simulink model "CM13_2024a_MachE_for_UA_HIL"  (R2024a)
settings: Solver=ode1  StartTime=0.0  StopTime=Inf  FixedStep=0.001  RelTol=1e-3  EnableMultiTasking=on
PreLoadFcn:
  | % if ~length(which('cmcmd')), cmenv; end
PostLoadFcn:
  | if any(exist('dsrtsu_mdlpostloadfcn', 'file') ~= 0), dsrtsu_mdlpostloadfcn('Execute', bdroot); end
InitFcn:
  | , if any(exist('rtifpga_mdlclblib', 'file') ~= 0), rtifpga_mdlclblib('Init', bdroot); end,
  | , if any(exist('dsmpb_private', 'file') ~= 0), dsmpb_private('dsmpb_mdlclblib', 'Init', bdroot); end,
values from neighbouring files (symbols this model uses):
  CoastDown =     [Run_Simulink.mat]
  limitedMCT =     [Run_Simulink.mat]
  MCT =     [Run_Simulink.mat]
  pMCT =     [Run_Simulink.mat]
  RealSimPara =     [Run_Simulink.mat]
  Ref_speed = [13 13.007895099 13.015778396 13.023649891 13.031509584 13.039357475 13.047193564 13.055017851 13.062830336 13.070631019 13.0784199 13.086196979 ... (2669 elements, 2669x1)]    [Ref_speed_and_time.mat]
  Ref_time = [0 0.01 0.02 0.03 0.04 0.05 0.06 0.07 0.08 0.09 0.1 0.11 ... (2669 elements, 2669x1)]    [Ref_speed_and_time.mat]
  US06 =     [Run_Simulink.mat]
undefined symbols (not defined in the file or in its folder): AccelCmd, ActTqLF_Nm_, ActTqLR_Nm_, ActTqRF_Nm_, ActTqRR_Nm_, BattChargeLimitMaxPwr, BattChargeLimitSocBpts, BattChargeLimitTbl, BattChrgCapcty, BattDischargeLimitSocBpts, BattDischargeLimitTbl, BattDischargeMaxPwr, BattNumCellsParallel, BattNumCellsSeries, BattOpenVoltCapBpts, BattOpenVoltTbl, BattResistSocBpts, BattResistTbl, BattResistTempBpts, BrakeMaxPrs, BrakeMaxTrq, ChassisDistCg2FrontAxle, ChassisDistCg2RearAxle, ChassisVehMass, CltchCmd, DecelCmd, DiffRatio, DiscIntNeverNeededParam, EnvGravCnst, EnvPrs, EnvTemp, FuelSpecificGrav, GearCmd, h, InitStates, lgSw, MtrEffSpdBpts, MtrEffTbl, MtrEffTrqBpts, MtrPwrMax, MtrTrqMax, planned_speed, planned_time, ref_speed, ref_time, rticanmm_blockfcn, rticanmm_initfcn, SteeringCmd, SupvsryCtrlRegenBrkCutOffTbl, SupvsryCtrlRegenSpdBpts, TestScnrioCycleNum, VEH
libraries: simulink x264, VSIGenLib x262, etargetslib x201, dsmpblib x161, CarMaker4SL x142, rtimmsu_dsrtlib x32, vehdynlibtire x24, autolibshared x19, vehdynlibsuspension x14, vehdynlibtirecommon x14, autolibutils x10, VsrLibWheel x8
(part 8 of 48)

== system CM13_2024a_MachE_for_UA_HIL/CarMaker/IPG Vehicle/Rototest and ORNL Interface ==
  note: CM driver = 0
      | Simulink driver = 1
  note: rad/s
  CarTrqT2W : Inport
  UDP Input : Inport  Port=2
  BRAKE_PRESSED : Inport  Port=3
  vehSpeedKph : Inport  Port=4
  1/tireRadius : Gain  Gain=1/0.3232
  ChargingMode : Constant  Value=0
  CmdSpeed (mph) : Constant  Value=0
  Constant : Constant  Value=3000
  DriverSwitch : Constant  Value=0
  DummyPT : Subsystem
  Format CM Powertrain Signals : Subsystem
  From Rototest : Subsystem
  Gain1 : Gain  Commented=on  Gain=3.6
  Get Wheel Spd Cmd Based on Wheel Dynamics : Subsystem
  Multiport Switch : MultiPortSwitch  DataPortOrder=Zero-based contiguous  Inputs=2  zeroidx=on  SaturateOnIntegerOverflow=off  InputSameDT=off
  Multiport Switch1 : MultiPortSwitch  DataPortOrder=Zero-based contiguous  Inputs=2  zeroidx=on  SaturateOnIntegerOverflow=off  InputSameDT=off
  Read CM Dict : CarMaker4SL/Read CM Dict  Commented=on  xname=Car.v  xsync=off  xstime=Continuous
  RotoTrqPreprocess : Subsystem
  Subsystem2 : Subsystem
  Terminator2 : Terminator
  To Rototest with Band-Aid : Subsystem
  mph2m/s : Gain  Gain=0.44704
  BrakeUpd : Outport
  Powertrain Out : Outport  Port=2
  DataSend : Outport  Port=3
  AutoMasterSW_Signal : Outport  Port=4
  wires:
  From Rototest/2(AxlTrq) -> RotoTrqPreprocess/1(AxleTrqRaw), Subsystem2/1(AxlTorq)
  From Rototest/1(SpdAct) -> To Rototest with Band-Aid/5(SpdAct), Terminator2/1  "SpdAct"
  [MaxRegen] -> Get Wheel Spd Cmd Based on Wheel Dynamics/4(MaxRegen)
  [MaxRegen] -> Format CM Powertrain Signals/4(MaxRegen)
  Get Wheel Spd Cmd Based on Wheel Dynamics/1(WhlSpdCmd) -> To Rototest with Band-Aid/1(SpeedCmd_rps), DummyPT/1(WhlSpeedIn), Multiport Switch1/2  "WhlSpdCmd"
  Multiport Switch/1 -> Get Wheel Spd Cmd Based on Wheel Dynamics/3(AxlTrq)
  RotoTrqPreprocess/2(AxleTrqVeh) -> Format CM Powertrain Signals/3(AxlTrq), Multiport Switch/2
  RotoTrqPreprocess/1(AxleTrqRoto) -> [AxlTrqRoto]
  [AxlTrqRoto] -> To Rototest with Band-Aid/2(AxleTrq_roto_Nm)
  Format CM Powertrain Signals/1(PowerTrainOutIdeal) -> Powertrain Out/1
  DriverSwitch/1 -> Multiport Switch/1
  UDP Input/1 -> From Rototest/1(Input)
  Subsystem2/1(BrakeUpd) -> BrakeUpd/1, Get Wheel Spd Cmd Based on Wheel Dynamics/1(BrakingTorques), Format CM Powertrain Signals/1(BrakingTorques)
  CarTrqT2W/1 -> Get Wheel Spd Cmd Based on Wheel Dynamics/2(Trq_T2W)
  DummyPT/1(WheelTorqueOut) -> Multiport Switch/3
  To Rototest with Band-Aid/1(Out1) -> DataSend/1  "DataSend"
  Constant/1 -> [MaxRegen]
  BRAKE_PRESSED/1 -> Get Wheel Spd Cmd Based on Wheel Dynamics/5(brkPressed), To Rototest with Band-Aid/3(BRAKE_PRESSED)
  Multiport Switch1/1 -> Format CM Powertrain Signals/2(RotoWheelSpd)
  ChargingMode/1 -> Multiport Switch1/1
  CmdSpeed (mph)/1 -> mph2m/s/1
  1/tireRadius/1 -> Multiport Switch1/3
  mph2m/s/1 -> 1/tireRadius/1
  Read CM Dict/1 -> Gain1/1  "VehSpd"
  vehSpeedKph/1 -> Get Wheel Spd Cmd Based on Wheel Dynamics/6(vehSpd), To Rototest with Band-Aid/4(Vehicle_Speed_kph)  "VehSpdKph"
  To Rototest with Band-Aid/2(AutoMasterSW_Signal) -> AutoMasterSW_Signal/1

== system CM13_2024a_MachE_for_UA_HIL/CarMaker/IPG Vehicle/SUMO Spd ==
  note: if no/broken tcp connection, 0 speed, otherwise use tcp data
  note: TCP Connection State
      | Server :
      | 2: The function block listens for connection requests of a TCP client
      | 3: The function block is connected to a TCP client
      | 4: The connection to the TCP client has been broken. The function block restarts the listen process.
      |
      | Client:
      | 0: The function block is not connected
      | 1: The function block tries to connect a TCP server
      | 3: The function block is connected to a TCP server
      | 4: The function block retries to connect a TCP server after the connection could not be established
      | 5: The function block cannot connect to the TCP server.
  note: Must use TCP as a server in dSPACE!!!!!!!!!!!!!!
  note: Here send and receive need to be modulated, otherwise sumo will stuck
  note: Source code from Yunli. It will use simlink time and sumo time to determin if sned or not
  0_Spd : Constant  Value=0
  Add : Sum
  Add1 : Sum
  Bus Selector : BusSelector  OutputSignals=NearPnt ds x,NearPnt ds y
  Bus Selector1 : BusSelector  OutputSignals=NearPnt dv x,NearPnt dv y
  Bus Selector2 : BusSelector  OutputSignals=dtct
  Clock : Clock
  Clock1 : Clock
  Connection State : Scope
  Constant : Constant  Value=1024
  Constant1 : Constant  Value=99999
  Constant2 : Constant  Value=zeros(1004,1);  OutDataTypeStr=uint8
  Data Type Conversion1 : DataTypeConversion  OutDataTypeStr=double  SaturateOnIntegerOverflow=off  RndMeth=Floor
  Data Type Conversion2 : DataTypeConversion  SaturateOnIntegerOverflow=off  RndMeth=Floor
  Data Type Conversion3 : DataTypeConversion  OutDataTypeStr=double  SaturateOnIntegerOverflow=off  RndMeth=Floor
  Data Type Conversion4 : DataTypeConversion  OutDataTypeStr=double  SaturateOnIntegerOverflow=off  RndMeth=Floor
  Defloater{,1..4} (5 alike) : VSIGenLib/Defloater  SystemSampleTime=-1  VariantActivationTime=update diagram  AllowFlexibleInterface=on  Latency=0  AutoFrameSizeCalculation=off
  DetectedDS : Scope
  DetectedDV : Scope
  Ethernet RefSpd1 : dsmpblib/Data Inport  Priority=10000
      settings: SourceProductName=dSPACE Model Interface Package for Simulink (MIPS)
  Floater : VSIGenLib/Floater  SystemSampleTime=-1  VariantActivationTime=update diagram  AllowFlexibleInterface=on  Latency=0  AutoFrameSizeCalculation=off
  Floater1 : VSIGenLib/Floater  SystemSampleTime=-1  VariantActivationTime=update diagram  AllowFlexibleInterface=on  Latency=0  AutoFrameSizeCalculation=off
  MATLAB System : MATLABSystem  System=RealSimTrigger  initialSpeed=0  speedLookAheadHorizon=1  speedUpperBound=30  smoothWindow=5  SimulateUsing=Code generation
      mask Type: RealSimTrigger
      mask Display:
      | disp('RealSimTrigger');
      | port_label('input',1,'simulationTime');
      | port_label('input',2,'connectionState');
      | port_label('input',3,'timeReceive');
      | port_label('input',4,'speedReceive');
      | port_label('input',5,'speedActual');
      | port_label('output',1,'speedLookAhead');
      | port_label('output',2,'accelerationDesired');
      | port_label('output',3,'timeSimulator');
      | port_label('output',4,'timeStepSimulator');
      | port_label('output',5,'timeStepTrigger');
      | port_label('output',6,'RealSimDelay');
  Manual Switch : ManualSwitch  CurrentSetting=0
  Math Function{,1..3} (4 alike) : Math  Operator=square
  Memory : Memory  InheritSampleTime=on
  Memory1 : Memory  InheritSampleTime=on
  Multiport Switch1 : MultiPortSwitch  DataPortOrder=Specify indices  Inputs=2  DataPortIndices={2,3,4}  SaturateOnIntegerOverflow=off  InputSameDT=off
  Mux : Mux  Inputs=6
  Object Sensor : CarMaker4SL/Sensors/Object Sensor  xname=RadarL  xstime=Continuous
      settings: SourceProductName=CarMaker4SL
  Object Sensor Object : CarMaker4SL/Sensors/Object Sensor Object  xname=INPORT  ximode=Observed Objects  xstime=Continuous
      settings: SourceProductName=CarMaker4SL
  Pulse Generator : DiscretePulseGenerator  PulseType=Time based  Period=0.1
  Read CM Dict : CarMaker4SL/Read CM Dict  xname=Car.v  xsync=off  xstime=Continuous
  Read CM Dict1 : CarMaker4SL/Read CM Dict  Commented=on  xname=Sensor.Object.RadarL.relvTgt.NearPnt.dv.x  xsync=off  xstime=Continuous
  Read CM Dict2 : CarMaker4SL/Read CM Dict  Commented=on  xname=Sensor.Object.RadarL.relvTgt.NearPnt.dv.y  xsync=off  xstime=Continuous
  Read CM Dict3 : CarMaker4SL/Read CM Dict  Commented=on  xname=Sensor.Object.RadarL.relvTgt.NearPnt.ds.y  xsync=off  xstime=Continuous
  Read CM Dict4 : CarMaker4SL/Read CM Dict  Commented=on  xname=Sensor.Object.RadarL.relvTgt.NearPnt.ds.x  xsync=off  xstime=Continuous
  Read CM Dict5 : CarMaker4SL/Read CM Dict  xname=Car.v  xsync=off  xstime=Continuous
  Read CM Dict6 : CarMaker4SL/Read CM Dict  xname=Car.atHori  xsync=off  xstime=Continuous
  Receive State : Scope
  Receive [TCP Ref Speed]1 : dsmpblib/Data Inport  Priority=10000
      settings: SourceProductName=dSPACE Model Interface Package for Simulink (MIPS)
  Selector1 : Selector  InputPortWidth=1024  IndexOptions=Index vector (dialog)  Indices=[4 3 2 1]  OutputSizes=1
  Selector4 : Selector  InputPortWidth=1024  IndexOptions=Index vector (dialog)  Indices=[8 7 6 5]  OutputSizes=1
  Square Root : Sqrt
  Square Root1 : Sqrt
  Status/Control [TCP Ref Speed] : dsmpblib/Data Inport  Priority=10000
      settings: SourceProductName=dSPACE Model Interface Package for Simulink (MIPS)
  Switch : Switch  Criteria=u2 > Threshold  SaturateOnIntegerOverflow=off  InputSameDT=off
  Switch1 : Switch  Criteria=u2 > Threshold  SaturateOnIntegerOverflow=off  InputSameDT=off
  Terminator{,1..9} (10 alike) : Terminator
  Transmit_In [TCP Ref Speed]1 : dsmpblib/Data Inport  Priority=10000
      settings: SourceProductName=dSPACE Model Interface Package for Simulink (MIPS)
  dSPACE TCP Out : Subsystem
  isDetected : Scope
  uint8 (unsigned 8) 4 : etargetslib/Byte Pack  datatypes={'uint8'}  byteAlign=1
  SUMO_spd : Outport
  wires:
  Receive [TCP Ref Speed]1/3 -> Terminator3/1
  Floater/1 -> Data Type Conversion1/1
  Selector4/1 -> Floater/1
  Receive [TCP Ref Speed]1/2 -> Receive State/1, Terminator4/1  "SumoTCP_Rec_stat"
  Receive [TCP Ref Speed]1/4 -> Terminator5/1
  Data Type Conversion1/1 -> MATLAB System/4, Multiport Switch1/3
  Clock/1 -> Defloater/1
  Defloater/1 -> Mux/1
  Constant2/1 -> uint8 (unsigned 8) 4/1
  Transmit_In [TCP Ref Speed]1/1 -> Terminator2/1
  Transmit_In [TCP Ref Speed]1/2 -> Terminator1/1
  Ethernet RefSpd1/1 -> Terminator6/1
  Data Type Conversion2/1 -> dSPACE TCP Out/1(ByteSend)
  Mux/1 -> Data Type Conversion2/1
  Status/Control [TCP Ref Speed]/2 -> Terminator7/1
  Status/Control [TCP Ref Speed]/3 -> Terminator8/1
  Status/Control [TCP Ref Speed]/1 -> [ConnectionState], Connection State/1
  Constant/1 -> dSPACE TCP Out/2(nMsgSend)
  Pulse Generator/1 -> Manual Switch/1
  [ConnectionState] -> Data Type Conversion4/1
  Clock1/1 -> MATLAB System/1
  Read CM Dict/1 -> MATLAB System/5  "VehSpd"
  Manual Switch/1 -> dSPACE TCP Out/3(sendTrigger)
  MATLAB System/5 -> Manual Switch/2  "RS_timeStepTrigger"
  Receive [TCP Ref Speed]1/1 -> Selector1/1, Selector4/1
  Floater1/1 -> Data Type Conversion3/1
  Selector1/1 -> Floater1/1
  Data Type Conversion3/1 -> MATLAB System/3  "Sumo_timeReceive"
  Data Type Conversion4/1 -> MATLAB System/2
  MATLAB System/4 -> Terminator/1  "RS_timeStepSimulator"
  MATLAB System/3 -> Terminator9/1  "RS_timeSimulator"
  Bus Selector/1 -> Math Function/1  "<NearPnt ds x>"
  Bus Selector/2 -> Math Function1/1  "<NearPnt ds y>"
  Bus Selector1/2 -> Math Function3/1  "<NearPnt dv y>"
  Bus Selector1/1 -> Math Function2/1  "<NearPnt dv x>"
  Math Function/1 -> Add/1
  Math Function1/1 -> Add/2
  Add/1 -> Square Root/1
  Add1/1 -> Square Root1/1
  Math Function2/1 -> Add1/1
  Math Function3/1 -> Add1/2
  Square Root/1 -> DetectedDS/1, Defloater1/1
  Square Root1/1 -> DetectedDV/1, Defloater2/1
  Defloater1/1 -> Mux/2
  Defloater2/1 -> Mux/3
  uint8 (unsigned 8) 4/1 -> Mux/6
  Defloater3/1 -> Mux/4
  Read CM Dict5/1 -> Defloater3/1  "VehSpd"
  Object Sensor/1 -> Object Sensor Object/1
  Object Sensor Object/4 -> Switch1/1, Switch/1
  Object Sensor Object/3 -> Bus Selector2/1
  Bus Selector2/1 -> Switch1/2, isDetected/1, Switch/2  "<dtct>"
  Memory/1 -> Switch/3
  Memory1/1 -> Switch1/3
  Defloater4/1 -> Mux/5
  Read CM Dict6/1 -> Defloater4/1
  Constant1/1 -> Object Sensor Object/2
  Switch/1 -> Memory/1
  Switch1/1 -> Memory1/1
  Object Sensor Object/5 -> Bus Selector1/1, Bus Selector/1
  [ConnectionState] -> Multiport Switch1/1
  Multiport Switch1/1 -> SUMO_spd/1
  0_Spd/1 -> Multiport Switch1/4, Multiport Switch1/2

== system CM13_2024a_MachE_for_UA_HIL/CarMaker/IPG Vehicle/Steering Angle HIL ==
  SteerAngCAN_in : Inport
  VhclCtrlBus : Inport  Port=2
  Bus Creator : BusCreator  Inputs=5
  Bus Selector : BusSelector  Commented=on  OutputSignals=VhclCtrl Steering Ang,VhclCtrl Steering AngVel,VhclCtrl Steering AngAcc,VhclCtrl Steering Trq,VhclCtrl Steering SteerByTrq
  Steering Override : Subsystem
  VhclCtrlBus_override : Outport
  wires:
  Bus Selector/5 -> Bus Creator/5  "<VhclCtrl Steering SteerByTrq>"
  Bus Creator/1 -> VhclCtrlBus_override/1
  Bus Selector/4 -> Bus Creator/4  "<VhclCtrl Steering Trq>"
  VhclCtrlBus/1 -> Bus Selector/1
  Bus Selector/2 -> Bus Creator/2  "<VhclCtrl Steering AngVel>"
  Bus Selector/3 -> Bus Creator/3  "<VhclCtrl Steering AngAcc>"
  Bus Selector/1 -> Steering Override/2(<VhclCtrl Steering Ang>)  "<VhclCtrl Steering Ang>"
  Steering Override/1(VhclCtrl Steering Ang) -> Bus Creator/1
  SteerAngCAN_in/1 -> Steering Override/1(SteerAngCAN_in)

== system CM13_2024a_MachE_for_UA_HIL/CarMaker/IPG Vehicle/Subsystem ==
  note: With tire radius correction of 1.14
  <VehSpd> : Inport
  Abs : Abs  SaturateOnIntegerOverflow=off
  Constant4 : Constant  Value=0  SampleTime=-1
  Gain5 : Gain  Gain=3.6*1.08
  Switch : Switch  Threshold=0.1  SaturateOnIntegerOverflow=off  InputSameDT=off
  Transfer Fcn12 : TransferFcn  Denominator=[0.02 1]
  VehSpdKph : Outport
  wires:
  Constant4/1 -> Switch/3
  Abs/1 -> Switch/2
  <VehSpd>/1 -> Transfer Fcn12/1
  Transfer Fcn12/1 -> Abs/1, Switch/1
  Gain5/1 -> VehSpdKph/1  "VehSpdKph"
  Switch/1 -> Gain5/1

== system CM13_2024a_MachE_for_UA_HIL/CarMaker/VehicleControl/CreateBus Vhcl.Misc ==
  In1 : Inport
  BusCreator : BusCreator  Inputs=11
  Demux : Demux  Outputs=11
      settings: DisplayOption=none
  Out1 : Outport  VectorParamsAs1DForOutWhenUnconnected=off
  wires:
  Demux/11 -> BusCreator/11  "Vhcl Wind_vel_0 z"
  Demux/10 -> BusCreator/10  "Vhcl Wind_vel_0 y"
  Demux/9 -> BusCreator/9  "Vhcl Wind_vel_0 x"
  Demux/8 -> BusCreator/8  "Vhcl Trq_DL2BdyEng y"
  Demux/7 -> BusCreator/7  "Vhcl Trq_DL2BdyEng x"
  Demux/6 -> BusCreator/6  "Vhcl Trq_DL2Bdy1B z"
  Demux/5 -> BusCreator/5  "Vhcl Trq_DL2Bdy1B y"
  Demux/4 -> BusCreator/4  "Vhcl Trq_DL2Bdy1B x"
  Demux/3 -> BusCreator/3  "Vhcl Trq_DL2Bdy1 z"
  Demux/2 -> BusCreator/2  "Vhcl Trq_DL2Bdy1 y"
  Demux/1 -> BusCreator/1  "Vhcl Trq_DL2Bdy1 x"
  In1/1 -> Demux/1
  BusCreator/1 -> Out1/1

== system CM13_2024a_MachE_for_UA_HIL/CarMaker/VehicleControl/CreateBus Vhcl.Wheel.In ==
  In1 : Inport
  Bus Creator1 : BusCreator  Inputs=12
  Demux1 : Demux  Outputs=12
      settings: DisplayOption=none
  Out1 : Outport  VectorParamsAs1DForOutWhenUnconnected=off
  wires:
  Demux1/12 -> Bus Creator1/12  "Vhcl Wheel RR rotv"
  Demux1/11 -> Bus Creator1/11  "Vhcl Wheel RR Trq_DL2WC"
  Demux1/10 -> Bus Creator1/10  "Vhcl Wheel RR Trq_B2WC"
  Demux1/9 -> Bus Creator1/9  "Vhcl Wheel RL rotv"
  Demux1/8 -> Bus Creator1/8  "Vhcl Wheel RL Trq_DL2WC"
  Demux1/7 -> Bus Creator1/7  "Vhcl Wheel RL Trq_B2WC"
  Demux1/6 -> Bus Creator1/6  "Vhcl Wheel FR rotv"
  Demux1/5 -> Bus Creator1/5  "Vhcl Wheel FR Trq_DL2WC"
  Demux1/4 -> Bus Creator1/4  "Vhcl Wheel FR Trq_B2WC"
  Demux1/3 -> Bus Creator1/3  "Vhcl Wheel FL rotv"
  In1/1 -> Demux1/1
  Bus Creator1/1 -> Out1/1
  Demux1/2 -> Bus Creator1/2  "Vhcl Wheel FL Trq_DL2WC"
  Demux1/1 -> Bus Creator1/1  "Vhcl Wheel FL Trq_B2WC"

== system CM13_2024a_MachE_for_UA_HIL/CarMaker/VehicleControl/CreateBus VhclCtrl ==
  In : Inport
  Gas : Inport  Port=2
  Brake : Inport  Port=3
  BusCreator : BusCreator  Inputs=29
  Demux : Demux  Outputs=29
      settings: DisplayOption=none
  Terminator : Terminator
  Terminator1 : Terminator
  Out : Outport
  wires:
  In/1 -> Demux/1
  BusCreator/1 -> Out/1
  Demux/1 -> BusCreator/1  "VhclCtrl SST"
  Demux/2 -> BusCreator/2  "VhclCtrl Key"
  Demux/3 -> BusCreator/3  "VhclCtrl UserSignal0"
  Demux/4 -> BusCreator/4  "VhclCtrl UserSignal1"
  Demux/5 -> BusCreator/5  "VhclCtrl UserSignal2"
  Demux/6 -> BusCreator/6  "VhclCtrl UserSignal3"
  Demux/7 -> BusCreator/7  "VhclCtrl UserSignal4"
  Demux/8 -> BusCreator/8  "VhclCtrl GearNo"
  Demux/9 -> BusCreator/9  "VhclCtrl SelectorCtrl"
  Demux/10 -> Terminator/1  "VhclCtrl Brake"
  Demux/11 -> BusCreator/11  "VhclCtrl BrakePark"
  Demux/12 -> BusCreator/12  "VhclCtrl Clutch"
  Demux/13 -> Terminator1/1  "VhclCtrl Gas"
  Demux/14 -> BusCreator/14  "VhclCtrl Steering Ang"
  Demux/15 -> BusCreator/15  "VhclCtrl Steering AngVel"
  Demux/16 -> BusCreator/16  "VhclCtrl Steering AngAcc"
  Demux/17 -> BusCreator/17  "VhclCtrl Steering Trq"
  Demux/18 -> BusCreator/18  "VhclCtrl Lights LowBeam"
  Demux/19 -> BusCreator/19  "VhclCtrl Lights HighBeam"
  Demux/20 -> BusCreator/20  "VhclCtrl Lights Daytime"
  Demux/21 -> BusCreator/21  "VhclCtrl Lights ParkL"
  Demux/22 -> BusCreator/22  "VhclCtrl Lights ParkR"
  Demux/23 -> BusCreator/23  "VhclCtrl Lights IndL"
  Demux/24 -> BusCreator/24  "VhclCtrl Lights IndR"
  Demux/25 -> BusCreator/25  "VhclCtrl Lights FogFrontL"
  Demux/26 -> BusCreator/26  "VhclCtrl Lights FogFrontR"
  Demux/27 -> BusCreator/27  "VhclCtrl Lights FogRear"
  Demux/28 -> BusCreator/28  "VhclCtrl Lights Brake"
  Demux/29 -> BusCreator/29  "VhclCtrl Lights Reverse"
  Gas/1 -> BusCreator/13
  Brake/1 -> BusCreator/10

== system CM13_2024a_MachE_for_UA_HIL/CarMaker/VehicleControl/CreateBus VhclCtrl.PT ==
  In1 : Inport
  BusCreator1 : BusCreator  Inputs=12
  Demux1 : Demux  Outputs=12
      settings: DisplayOption=none
  Out1 : Outport  VectorParamsAs1DForOutWhenUnconnected=off
  wires:
  Demux1/12 -> BusCreator1/12  "VhclCtrl Brake"
  Demux1/11 -> BusCreator1/11  "VhclCtrl Gas"
  Demux1/10 -> BusCreator1/10  "VhclCtrl Clutch"
  Demux1/9 -> BusCreator1/9  "VhclCtrl SelectorCtrl"
  Demux1/8 -> BusCreator1/8  "VhclCtrl GearNo"
  Demux1/7 -> BusCreator1/7  "VhclCtrl UserSignal4"
  Demux1/6 -> BusCreator1/6  "VhclCtrl UserSignal3"
  Demux1/5 -> BusCreator1/5  "VhclCtrl UserSignal2"
  Demux1/4 -> BusCreator1/4  "VhclCtrl UserSignal1"
  Demux1/3 -> BusCreator1/3  "VhclCtrl UserSignal0"
  Demux1/2 -> BusCreator1/2  "VhclCtrl Key"
  Demux1/1 -> BusCreator1/1  "VhclCtrl SST"
  In1/1 -> Demux1/1
  BusCreator1/1 -> Out1/1

== system CM13_2024a_MachE_for_UA_HIL/CarMaker/VehicleControl/CreateBus VhclCtrl.Steering ==
  In1 : Inport
  Bus Creator : BusCreator  Inputs=5
  Demux : Demux  Outputs=5
      settings: DisplayOption=none
  Out1 : Outport  VectorParamsAs1DForOutWhenUnconnected=off
  wires:
  In1/1 -> Demux/1
  Bus Creator/1 -> Out1/1
  Demux/1 -> Bus Creator/1  "VhclCtrl Steering Ang"
  Demux/5 -> Bus Creator/5  "VhclCtrl Steering SteerByTrq"
  Demux/3 -> Bus Creator/3  "VhclCtrl Steering AngAcc"
  Demux/2 -> Bus Creator/2  "VhclCtrl Steering AngVel"
  Demux/4 -> Bus Creator/4  "VhclCtrl Steering Trq"

== system CM13_2024a_MachE_for_UA_HIL/CarMaker_new/IPG Vehicle/AEB Flag ==
  Bus Selector : BusSelector  OutputSignals=ACCDATA_2.CmbbBrkDecel_A_Rq,PowertrainData_10.TrnRng_D_Rq,PowertrainData_10.TrnPrkSys_D_Actl,PowertrainData_10.GearPos_D_Actl,PowertrainData_10.GearLvr_D_ActlDrv,Battery_Traction_2_FD1.BattTrac_U2_Actl,Battery_Traction_2_FD1.BattTrac_I2_Actl
  Gain{,1..4,6} (6 alike) : Gain
  RTICANMM ControllerSetup : Subsystem  InitFcn=rticanmm_blockfcn('InitFcn', 'CANnedySetup', gcb)  ClipboardFcn=rticanmm_blockfcn('ClipboardFcn', 'CANnedySetup', gcb)  mask(RTICANMM){DSProperties=struct('RTI',struct('Version',uint32(1),'BlockType',struct('isSLSource',uint8(1),'isSLSink',uint8(1),'isHWSource',uint8(0),'isHWSink',uint8(0),'isSetup',uint8(0),'isInline',uint8(1),'isNonInline',uint8(0),'isInterrupt',uint8(0),'isChannelwise',uint8(0)),'IOBoardType','RTICANMM','UnitType','RTICANMM','Identifier','BUSSETUP','DialogType','SL','BlockSet','RTICANMM','SlaveProcessor','CAN')), CANMMProperties=struct('cannedy',struct('data',struct('options',struct('controllername','MachE_FD1','controllernameautomatic',0,'loglevel','0','checkrealtime',0,'checkchangebaudrate',0,'sampletime','1.000','CANControllerStatus',1,'NumberofStuffErr',0,'NumberofFormErr',0,'NumberofAckErr',0,'NumberofBit0Err',1,'NumberofsuccrecRX',0,'Numberofsuccsent',0,'NumberofBit1Err',1,'NumberofCRCErr',1,'NumberoflostRX',0,'Busoff',0,'Busload',0,'OperationPending',0,'TxRetryCount',3,'addtrcexclusion',true,'cannavigator',struct('checkmonitoring',0,'checkinternmonitoring',0),'show_usrtrc',0,'use_usrtrc',0,'checkchangebaudrateFD',0,'errorframegeneration',0,'efgenabled',1),'modelroot','C:\GitDev\Yunli\FordMachE\HIL-Operation\src_cm4sl','generalsettings',struct('setupdata',struct('board','DS2671','boardno',1,'channelno',1,'Type','STD','transceiver',['ISO 11898-2 HIGH SPEED CAN'],'busconfig',[],'feedthrough','false','resistance',struct('r120',1,'roff',0,'r16',0,'r10',1),'baudrate','500','Frequency',[24 36],'samplemode',1,'commChannelTJA1041',6,'config',struct('standard',1,'advanced',0,'register',struct('btr0','0xC0','btr1','0x6F','sp','70','sjw','v','tseg1','15','tseg2','6','brp','0','smpl','0','btr0_36','0x1','btr1_36','0x2D','sp_36','83','sjw_36','0','tseg1_36','12','tseg2_36','2','brp_36','1','smpl_36','0','btr0_64','0x3','btr1_64','0x2B','sp_64','81','sjw_64','0','tseg1_64','11','tseg2_64','2','brp_64','3','smpl_64','0')),'channelcfg',struct('INTENDISABLE','CAN_INT_DISABLE','intenable',0),'SETUPID','RTICANMM_MachE_FD1_ID','CONTROLLER_ID','CANMM_CTL_SETUP_MachE_FD1','mainblock_includefile','RTICANMM_SETUP_MachE_FD1','canfdenable',2,'canfdboardselected',1,'slotno',1,'moduletype','DS4342','baudrateFD','2000','samplePoint','80','samplePointFD','80','termination','TERMINATION_ON'),'filesettings',struct('destfolder',struct('Name','RTICANMM_FILES','Check',1),'buildfolder',struct('Name','.','Check',1))),'advanced',struct('options',ones(1,100)),'partialnetdata',struct('switchedon',0,'format','STD','idmask',['XXXXX XXXXXXXX XXXXXXXX XXXXXXXX'],'idcode','0','idfilter','0','datamaskused',0,'datalength','0','datamask','0x0000000000000000','partialnetworkenable',0)),'blk',['HIL_MachE_CM10/Vehicle Under Test/Vehicle/AEB Flag/RTICANMM' char(10) 'ControllerSetup'],'allgeneratedfiles',{{'C:\GitDev\Yunli\FordMachE\HIL-Operation\src_cm4sl\RTICANMM_FILES\RTICANMM_SETUP_MachE_FD1.c','C:\GitDev\Yunli\FordMachE\HIL-Operation\src_cm4sl\RTICANMM_FILES\RTICANMM_SETUP_MachE_FD1.h','c:\gitdev\yunli\fordmache\hil-operation\src_cm4sl\rticanmm_files\rticanmm_setup_mache_fd1.mexw64'}},'ismp',false,'BlockDataVersion','0.9.0','recreate',0,'CANnedyTag','MachE_FD1'),'CANnedynew',0,'CANnedySettings','MachE_FD1','GeneratedFiles',{{'C:\GitDev\Yunli\FordMachE\HIL-Operation\src_cm4sl\RTICANMM_FILES\RTICANMM_SETUP_MachE_FD1.c','C:\GitDev\Yunli\FordMachE\HIL-Operation\src_cm4sl\RTICANMM_FILES\RTICANMM_SETUP_MachE_FD1.h','c:\gitdev\yunli\fordmache\hil-operation\src_cm4sl\rticanmm_files\rticanmm_setup_mache_fd1.mexw64'}},'SFCN','RTICANMM_SETUP_MachE_FD1.c','HostService',struct('Tags',struct('DATA','RTICANMM_MonitorData','TimeStampGlobal','RTICANMM_MonitoringTimeStamp','TimeStampGlobalEnable','RTICANMM_MonitoringTimeStampEnable','Enable','CANMMMonitor_MachE_FD1','TimeStamp','MonitoringTimeStamp_MachE_FD1'),'DATA',struct('Length',18),'Info',struct('Desc',{'ID','Service','Data1','Data2','Data3','Data4','Data5','Data6','Data7','Data8','Data9','Data10','Data11','Data12','Data13','Data14','Data15','Data16'}),'Names',struct('TimeStampGlobal','TimeStamp','TimeStampGlobalEnable','TimeStamp_Enable','Enable','Monitoring_Enable','TimeStamp','Monitoring_TimeStamp'),'ChannelID',2)), CANMMType=CANnedySetup, CANMMFolder=C:\CM_Projects\UA_cave\CM13_proj\src_cm4dspace_realsim, CANMMDestFolder=RTICANMM_FILES, CANMMSettings=MachE_FD1, CANMMSFcn=RTICANMM_SETUP_MachE_FD1, CANMMBoard=DS2671, CANMMBoardNum=1, CANMMChannel=1}
      settings: AttributesFormatString=%<CANMMSettings>  CopyFcn=rticanmm_blockfcn('CopyFcn', 'CANnedySetup', gcb)  DeleteFcn=rticanmm_blockfcn('DeleteFcn', 'CANnedySetup', gcb)  ModelCloseFcn=rticanmm_blockfcn('ModelCloseFcn', 'CANnedySetup', gcb)  NameChangeFcn=rticanmm_blockfcn('NameChangeFcn', 'CANnedySetup', gcb)  OpenFcn=try, rticanmm_setup_gui('create',gcb); ; catch,errordlg({lasterr, '','Please check your RTI installation.'},['Error: ' upper(bdroot)], 'replace'); end  MoveFcn=rticanmm_blockfcn('MoveFcn', 'CANnedySetup', gcb)
      mask Help: eval('rticanmm_quickstart(''create'', gcb);', 'disp(lasterr);')
      mask Display:
      | disp('RTI CAN\nMultiMessage\nControllerSetup')
      | 
      | port_label('input', 1 , 'Variation')
      | port_label('input', 2 , 'Reset')
      | port_label('output', 1, 'Status')
      | port_label('output', 2, 'Bit 0 errors')
      | port_label('output', 3, 'Bit 1 errors')
      | port_label('output', 4, 'CRC errors')
  RTICANMM ControllerSetup1 : dsmpblib/Data Outport  Priority=-10000
      settings: SourceProductName=dSPACE Model Interface Package for Simulink (MIPS)
  RTICANMM MainBlock : Subsystem  InitFcn=rticanmm_blockfcn('InitFcn', 'CANnedy', gcb)  ClipboardFcn=rticanmm_blockfcn('ClipboardFcn', 'CANnedy', gcb)  mask(RTICANMM){DSProperties=struct('RTI',struct('Version',uint32(1),'BlockType',struct('isSLSource',uint8(1),'isSLSink',uint8(1),'isHWSource',uint8(0),'isHWSink',uint8(0),'isSetup',uint8(0),'isInline',uint8(1),'isNonInline',uint8(0),'isInterrupt',uint8(0),'isChannelwise',uint8(0)),'IOBoardType','RTICANMM','UnitType','RTICANMM','Identifier','Mainblock','DialogType','SL','BlockSet','RTICANMM','SlaveProcessor','CAN')), CANMMProperties=struct('RTICANMMVersion','24.1','RTICANMMVersionIntern','24.1.739338.0305092592','RTICANMMDate','02-May-2024','Settings','RTICANMM_MAIN_MachE_FD1','UserTracePath','','ModelPath','C:\CM_Projects\UA_cave\CM13_proj\src_cm4dspace_realsim','filesettings',struct('FileName','RTICANMM_FILES\FD1_CAN_CX727_BEV_MY21_DCV_V21.dbc','IsRelative',1,'ClusterId',1,'ClusterList',{{'default'}},'destfolder',struct('Name','RTICANMM_FILES','Check',1),'buildfolder',struct('Name','.','Check',1),'onlyfreerawcapture',0,'overlapping2variant',0,'canfdsupport',1,'shortestJ2container',1),'onlyfreerawcapture',0,'Board','DS2671','BoardNum','1','ChannelNum','1','Variation','1','SetupId','MachE_FD1','MARK',['1F517A29CDDA91C40D81A06F1A259F';'402B427622E552C8724AFAF21BAF37';'507793A5241270CA8226E0AA5FABF0';'03D6615B00574698D00C6826B10C14';'3DF76DA45C804484AF6D3344981453'],'date','08-May-2025','clock',['08.05.2025 17:13:54'],'recreate',0,'RTIVER','DSRT','j1939',0,'TRC',struct('include',1),'rtsupport',struct('XMLFile','C:\CM_Projects\UA_cave\CM13_proj\src_cm4dspace_realsim\RTICANMM_FILES\RTICANMM_MAIN_MachE_FD1.xml','DBCXML',struct('Path','C:\CM_Projects\UA_cave\CM13_proj\src_cm4dspace_realsim\RTICANMM_FILES\RTICANMM_MAIN_MachE_FD1_dbc.xml','support',1,'Name','FD1_CAN_CX727_BEV_MY21_DCV_V21.dbc','Date',['28-Mar-2023 17:18:35'],'Type','CAN_FD','DBCSupport','ON'))), CANMMType=CANnedy, CANMMUserTraceMerged=off, CANMMUserTracePath=, CANMMChannelNum=1, CANMMBoardNum=1, CANMMDestFolder=RTICANMM_FILES, CANMMFolder=., CANMMSetupId=MachE_FD1, CANMMsave2mat=['1F517A29CDDA91C40D81A06F1A259F';'402B427622E552C8724AFAF21BAF37';'507793A5241270CA8226E0AA5FABF0';'03D6615B00574698D00C6826B10C14';'3DF76DA45C804484AF6D3344981453'], CANMMName=MachE_FD1, CANMMSettings=RTICANMM_MAIN_MachE_FD1, CANMMIntermediateTag=RTICANMM_MAIN_MachE_FD1_intermediate, CANMMsfcnname=RTICANMM_MAIN_MachE_FD1}
      mask init:
      | rticanmm_initfcn(gcb, CANMMType, CANMMsfcnname)
      settings: AttributesFormatString=MachE_FD1[MachE_FD1]  CopyFcn=rticanmm_blockfcn('CopyFcn', 'CANnedy', gcb)  DeleteFcn=rticanmm_blockfcn('DeleteFcn', 'CANnedy', gcb)  ModelCloseFcn=rticanmm_blockfcn('ModelCloseFcn', 'CANnedy', gcb)  NameChangeFcn=rticanmm_blockfcn('NameChangeFcn', 'CANnedy', gcb)  OpenFcn=try, rticanmm_main_gui('create',gcb); ; catch,errordlg({lasterr, '','Please check your RTI installation.'},['Error: ' upper(bdroot)], 'replace'); end  MoveFcn=rticanmm_blockfcn('MoveFcn', 'CANnedy', gcb)
      mask Help: try, rticanmm_quickstart('create', gcb); catch ME, disp(ME.message);end
      mask Display:
      | disp(sprintf('RTI CAN\nMultiMessage\nMainBlock'))
      | port_label('output', 1, 'RX Data')
  Reset@RTICANMM ControllerSetup : Constant  Value=0  OutDataTypeStr=boolean
  Terminator{,1..6,9..11} (10 alike) : Terminator
  Variation@RTICANMM ControllerSetup : Constant  OutDataTypeStr=uint8
  Output : Outport
  wires:
  Variation@RTICANMM ControllerSetup/1 -> RTICANMM ControllerSetup/1(VariationInput)
  Reset@RTICANMM ControllerSetup/1 -> RTICANMM ControllerSetup/2(Reset)
  Bus Selector/1 -> Output/1  "<CmbbBrkDecel_A_Rq>"
  Bus Selector/2 -> Gain4/1  "<TrnRng_D_Rq>"
  RTICANMM ControllerSetup/1(BUS_STATE) -> Terminator1/1  "FD1_status"
  RTICANMM ControllerSetup/2(STATUS_BIT0_ERROR) -> Terminator2/1  "FD1_bit0_err"
  RTICANMM ControllerSetup/3(STATUS_BIT1_ERROR) -> Terminator3/1  "FD1_bit1_err"
  RTICANMM ControllerSetup/4(STATUS_CRC_ERROR) -> Terminator4/1  "FD1_CRC_err"
  Bus Selector/3 -> Gain3/1  "<TrnPrkSys_D_Actl>"
  Bus Selector/6 -> Gain2/1  "<BattTrac_U2_Actl>"
  Bus Selector/7 -> Gain1/1  "<BattTrac_I2_Actl>"
  Bus Selector/4 -> Gain/1  "<GearPos_D_Actl>"
  Bus Selector/5 -> Gain6/1  "<GearLvr_D_ActlDrv>"
  Gain4/1 -> Terminator6/1  "GearPos_D_Actl"
  Gain3/1 -> Terminator5/1  "GearPos_D_Actl"
  Gain/1 -> Terminator/1  "GearPos_D_Actl"
  Gain6/1 -> Terminator11/1  "GearLvr_D_Actl"
  Gain2/1 -> Terminator10/1  "BattTrac_U2_Actl"
  Gain1/1 -> Terminator9/1  "BattTrac_I2_Actl"
  RTICANMM MainBlock/1(RX_Data) -> Bus Selector/1

== system CM13_2024a_MachE_for_UA_HIL/CarMaker_new/IPG Vehicle/Actuation and Outputs ==
  note: Notes: 11.12.2024
      | Increased the brake limite from 50 to 80
  note: CarMaker Driver's Brake value is too mall to hold the Mach-E when parking
      | Instead of default value, we change it to 40%
  note: Pedal Control Selection
      | 1. Manual input
      | Gas: percentage
      | Brake: percentage
      | 2. From Driver bus commands
      | 3. CM Driver
      | 4. 0
  note: Temp added an Soft_AEB for testing
  note: Detect Rising signal from M_SW_signal.
      | When SW is turned on, reset AEB flag
  note: Driver Commands are [0,100] for both pedal and brake
  Driver Commands : Inport
  CM Driver Commands : Inport  Port=2
  AEB Cmd : Inport  Port=3
  A_M_SW_Sig : Inport  Port=4
  Veh_spd : Inport  Port=5
  AEB Flag Control : Logic  Operator=OR  IconShape=distinctive  AllPortsSameDT=off  OutDataTypeStr=boolean
  AND : Logic  IconShape=distinctive  AllPortsSameDT=off  OutDataTypeStr=boolean
  APP : Constant  Value=0
  AR_limit : Saturate  UpperLimit=100  LowerLimit=0
  Add : Sum
  Add1 : Sum
  BR_command_0to100 : Constant  Value=0
  BR_limit : Saturate  UpperLimit=80  LowerLimit=0
  Bus Creator : BusCreator  Inputs=2
  Bus Selector : BusSelector  Commented=on  OutputSignals=VhclCtrl Gas
  Bus Selector1 : BusSelector  OutputSignals=AccelPedalCmd
  Bus Selector2 : BusSelector  Commented=on  OutputSignals=VhclCtrl Brake
  Bus Selector3 : BusSelector  OutputSignals=BrakePedalCmd
  Compare To Constant : simulink/Logic and Bit Operations/Compare To Constant  relop=>=  const=3  OutDataTypeStr=boolean
  Compare To Constant1 : simulink/Logic and Bit Operations/Compare To Constant  relop=<=  const=0.1  OutDataTypeStr=boolean  ZeroCross=off
  Compare To Constant2 : simulink/Logic and Bit Operations/Compare To Constant  relop=<=  const=0.01  OutDataTypeStr=boolean  ZeroCross=off
  Constant : Constant  Value=0
  Constant1 : Constant  Value=0
  Constant2 : Constant  Value=0
  Detect Rise Positive : simulink/Logic and Bit Operations/Detect Rise Positive  vinit=0  OutDataTypeStr=boolean
  Gain : Gain  Gain=-1
  Gain1 : Gain  Gain=100
  Gain2 : Gain  Gain=100
  MOOG Brake Actuator : Subsystem
  Memory : Memory
  Min threshold for Brake switch : Constant  Value=0
  Multiport Switch1 : MultiPortSwitch  Inputs=4  SaturateOnIntegerOverflow=off  InputSameDT=off
  Multiport Switch2 : MultiPortSwitch  Inputs=4  SaturateOnIntegerOverflow=off  InputSameDT=off
  Pedal Reset : Constant  Value=0
  Pedal Robot Control Selection : Constant  Value=2
  Relational Operator : RelationalOperator  Operator=>  OutDataTypeStr=boolean  InputSameDT=off
  Soft_AEB : Constant  Value=0
  Switch : Switch  Criteria=u2 > Threshold  SaturateOnIntegerOverflow=off  InputSameDT=off
  Switch1 : Switch  Criteria=u2 > Threshold  SaturateOnIntegerOverflow=off  InputSameDT=off
  Switch4 : Switch  Criteria=u2 > Threshold  SaturateOnIntegerOverflow=off  InputSameDT=off
  Terminator : Terminator
  Vehicle Accel Pedal Voltage Output : Subsystem
  bped2br_N1 : Lookup_n-D  NumberOfTableDimensions=1  BreakpointsForDimension1=[0 0.1 0.2 100]  Table=[0 0 25 100]  InternalRulePriority=Speed  RndMeth=Simplest
  standstill brake [0,100] : Constant  Value=0.4
  BrakeSwitch : Outport  VectorParamsAs1DForOutWhenUnconnected=off
  CAVE_Driver : Outport  Port=2
  AEB_IS_Triggered : Outport  Port=3
  tag scope: BrakeDriver=global, CarlaSteer=global, GasDriver=global
  wires:
  Multiport Switch1/1 -> AR_limit/1
  APP/1 -> Multiport Switch1/2
  Bus Selector1/1 -> Multiport Switch1/3  "<AccelPedalCmd>"
  Gain2/1 -> Multiport Switch1/4
  Multiport Switch2/1 -> BR_limit/1
  Gain1/1 -> Multiport Switch2/4
  Driver Commands/1 -> Bus Selector3/1, Bus Selector1/1
  Pedal Robot Control Selection/1 -> Multiport Switch1/1, Multiport Switch2/1
  BR_command_0to100/1 -> Multiport Switch2/2
  CM Driver Commands/1 -> Bus Selector2/1, Bus Selector/1
  Bus Selector3/1 -> Multiport Switch2/3  "<BrakePedalCmd>"
  Min threshold for Brake switch/1 -> Relational Operator/2
  Relational Operator/1 -> BrakeSwitch/1  "BrakeSwitch"
  Constant/1 -> Multiport Switch1/5
  Constant1/1 -> [CarlaSteer], Multiport Switch2/5
  Bus Creator/1 -> CAVE_Driver/1
  BR_limit/1 -> MOOG Brake Actuator/1(Brake Pedal command [%]), Bus Creator/2, [BrakeDriver], Relational Operator/1  "BrakePedalCmd_pct"
  Switch/1 -> Vehicle Accel Pedal Voltage Output/1(APP_pct), [GasDriver], Bus Creator/1  "AccelPedalCmd_pct"
  Constant2/1 -> Switch1/1, Switch/1
  AEB Cmd/1 -> Gain/1
  Add/1 -> Memory/1
  Compare To Constant/1 -> Add1/2
  AR_limit/1 -> Switch/3  "AccelPedalCmd_pct"
  Gain/1 -> Compare To Constant/1
  Switch1/1 -> Add/2  "AccelPedalCmd_pct"
  Pedal Reset/1 -> AEB Flag Control/2
  Memory/1 -> AEB_IS_Triggered/1, Switch/2, Switch1/3
  A_M_SW_Sig/1 -> Detect Rise Positive/1
  Detect Rise Positive/1 -> AEB Flag Control/1
  AEB Flag Control/1 -> Terminator/1, Switch1/2  "AEB Flag Control"
  Soft_AEB/1 -> Add1/1
  Add1/1 -> Add/1
  standstill brake [0,100]/1 -> Switch4/1
  Compare To Constant1/1 -> AND/2
  Bus Selector2/1 -> Switch4/3  "<VhclCtrl Brake>"
  Switch4/1 -> Gain1/1  "BrakePedalPos_pct"
  Veh_spd/1 -> Compare To Constant1/1
  Bus Selector/1 -> Compare To Constant2/1, Gain2/1  "<VhclCtrl Gas>"
  Compare To Constant2/1 -> AND/1
  AND/1 -> Switch4/2

== system CM13_2024a_MachE_for_UA_HIL/CarMaker_new/IPG Vehicle/Brake ==
  note: When replacing the entire braking system,
      | be sure to disable the IPG brake model by using the brake
      | model 'Model Manager off' in the vehicle GUI.
  note: <Your model here>
  note: <Your model here>
  VehicleSimulationType : Inport
  Sync_In : Inport  Port=2
  Brake.IF.In : Inport  Port=3
  VhclCtrl.Brake : Inport  Port=4
  VhclCtrl.BrakeUpd : Inport  Port=5
  Brake : S-Function  FunctionName=CM_Sfun  Parameters='Brake'  SFunctionDeploymentMode=off  EnableBusSupport=off
  BrakeUpd : S-Function  FunctionName=CM_Sfun  Parameters='BrakeUpd'  SFunctionDeploymentMode=off  EnableBusSupport=off
  BusCreator1 : BusCreator  Inputs=16
  CreateBus Vhcl.Wheel.PT : Subsystem
  Demux : Demux  Outputs=16
      settings: DisplayOption=none
  Switch : Switch  Criteria=u2 > Threshold  SaturateOnIntegerOverflow=off  InputSameDT=off
  Sync_Out : Outport  VectorParamsAs1DForOutWhenUnconnected=off
  Vhcl.Wheel.PT : Outport  Port=2  VectorParamsAs1DForOutWhenUnconnected=off
  wires:
  Demux/16 -> BusCreator1/16  "Brake IF Trq_DriveSrc_trg d3"
  Demux/15 -> BusCreator1/15  "Brake IF Trq_DriveSrc_trg d2"
  Demux/14 -> BusCreator1/14  "Brake IF Trq_DriveSrc_trg d1"
  Demux/13 -> BusCreator1/13  "Brake IF Trq_DriveSrc_trg d0"
  Demux/12 -> BusCreator1/12  "Brake IF Trq_Reg_trg RR"
  Demux/11 -> BusCreator1/11  "Brake IF Trq_Reg_trg RL"
  Demux/10 -> BusCreator1/10  "Brake IF Trq_Reg_trg FR"
  Demux/9 -> BusCreator1/9  "Brake IF Trq_Reg_trg FL"
  Demux/8 -> BusCreator1/8  "Brake IF Trq_PB RR"
  Demux/7 -> BusCreator1/7  "Brake IF Trq_PB RL"
  Demux/6 -> BusCreator1/6  "Brake IF Trq_PB FR"
  Demux/5 -> BusCreator1/5  "Brake IF Trq_PB FL"
  Demux/4 -> BusCreator1/4  "Brake IF Trq_WB RR"
  Demux/3 -> BusCreator1/3  "Brake IF Trq_WB RL"
  Demux/2 -> BusCreator1/2  "Brake IF Trq_WB FR"
  Demux/1 -> BusCreator1/1  "Brake IF Trq_WB FL"
  Brake/2 -> Demux/1
  BrakeUpd/1 -> Sync_Out/1
  Brake/1 -> BrakeUpd/1  "Sync"
  Brake.IF.In/1 -> Brake/2
  VhclCtrl.Brake/1 -> Brake/3
  Sync_In/1 -> Brake/1
  BrakeUpd/2 -> CreateBus Vhcl.Wheel.PT/1(In)
  CreateBus Vhcl.Wheel.PT/1(Out) -> Vhcl.Wheel.PT/1
  VehicleSimulationType/1 -> Switch/2
  Switch/1 -> BrakeUpd/2
  BusCreator1/1 -> Switch/3
  VhclCtrl.BrakeUpd/1 -> Switch/1

== system CM13_2024a_MachE_for_UA_HIL/CarMaker_new/IPG Vehicle/CarAndTrailer ==
  Sync_In : Inport
  VhclCtrl.Steering : Inport  Port=2
  Vhcl.Wheel.In : Inport  Port=3
  Vhcl.Misc : Inport  Port=4
  CarAndTrailerUpd : Subsystem
  Forces : Subsystem
  Ground : Ground
  Kinematics : Subsystem
  Kinetics : Subsystem
  Steering : Subsystem
  Terminator : Terminator
  Terminator1 : Terminator
  Trailer : Subsystem
  Sync_Out : Outport  VectorParamsAs1DForOutWhenUnconnected=off
  Brake.IF.In : Outport  Port=2  VectorParamsAs1DForOutWhenUnconnected=off
  Car.Trq_T2W : Outport  Port=3
  wires:
  Trailer/9(Car.Hitch.FrcTrq) -> CarAndTrailerUpd/9(Car.Hitch.FrcTrq)
  Trailer/8(Vhcl.Wheel.RR) -> CarAndTrailerUpd/8(Vhcl.Wheel.RR)
  Trailer/7(Vhcl.Wheel.RL) -> CarAndTrailerUpd/7(Vhcl.Wheel.RL)
  Trailer/6(Vhcl.Wheel.FR) -> CarAndTrailerUpd/6(Vhcl.Wheel.FR)
  Trailer/5(Vhcl.Wheel.FL) -> CarAndTrailerUpd/5(Vhcl.Wheel.FL)
  Trailer/4(Vhcl.PoI) -> CarAndTrailerUpd/4(Vhcl.PoI)
  Trailer/3(Vhcl.Motion) -> CarAndTrailerUpd/3(Vhcl.Motion)
  Trailer/2(Vhcl.Steering) -> CarAndTrailerUpd/2(Vhcl.Steering)
  Trailer/1(Sync_Out) -> CarAndTrailerUpd/1(Sync_In)
  CarAndTrailerUpd/2(Brake.IF.In) -> Brake.IF.In/1
  CarAndTrailerUpd/1(Sync_Out) -> Sync_Out/1
  Vhcl.Misc/1 -> Terminator1/1
  Vhcl.Wheel.In/1 -> Terminator/1
  Kinetics/6(WheelCarrier.Misc) -> Trailer/6(WheelCarrier.Misc)
  Kinetics/5(Car.Trq_T2W) -> Car.Trq_T2W/1, Trailer/5(Car.Trq_T2W)
  Steering/2(Steer.IF) -> Kinematics/2(Steer.IF)
  Kinetics/4(Car.Fr1) -> Trailer/4(Car.Fr1)
  Kinetics/3(Car.Hitch) -> Trailer/3(Car.Hitch)
  Kinetics/2(Trailer.Load) -> Trailer/2(Trailer.Load)
  VhclCtrl.Steering/1 -> Steering/2(VhclCtrl.Steering)
  Sync_In/1 -> Steering/1(Sync_In)
  Steering/1(Sync_Out) -> Kinematics/1(Sync_In)
  Kinetics/1(Sync_Out) -> Trailer/1(Sync_In)
  Ground/1 -> CarAndTrailerUpd/10(Vhcl.Fr1A)
  Forces/11(FStabi_ext) -> Kinetics/11(FStabi_ext)
  Forces/10(FDamp_ext) -> Kinetics/10(FDamp_ext)
  Forces/9(FSpring_ext) -> Kinetics/9(FSpring_ext)
  Forces/8(TireRR_Out) -> Kinetics/8(TireRR.Out)
  Forces/7(TireRL_Out) -> Kinetics/7(TireRL.Out)
  Forces/6(TireFR_Out) -> Kinetics/6(TireFR.Out)
  Forces/5(TireFL_Out) -> Kinetics/5(TireFL.Out)
  Forces/4(Car.Load) -> Kinetics/4(Car.Load)
  Forces/2(Car.Virtual) -> Kinetics/2(Car.Virtual)
  Kinematics/6(lSpring) -> Forces/6(lSpring)
  Kinematics/7(vDamp) -> Forces/7(vDamp)
  Forces/3(Car.Aero) -> Kinetics/3(Car.Aero)
  Forces/1(Sync_Out) -> Kinetics/1(Sync_In)
  Kinematics/5(TireRR_In) -> Forces/5(TireRR_In)
  Kinematics/4(TireRL_In) -> Forces/4(TireRL_In)
  Kinematics/3(TireFR_In) -> Forces/3(TireFR_In)
  Kinematics/2(TireFL_In) -> Forces/2(TireFL_In)
  Kinematics/1(Sync_Out) -> Forces/1(Sync_In)
  Kinematics/8(lStabi) -> Forces/8(lStabi)
  Forces/12(FBuf_ext) -> Kinetics/12(FBuf_ext)
  Kinematics/9(lBuf) -> Forces/9(lBuf)

== system CM13_2024a_MachE_for_UA_HIL/CarMaker_new/IPG Vehicle/DARTS ConfigDesk Control ==
  Enable : Inport
  Range : Inport  Port=2
  Speed : Inport  Port=3
  Gain : Inport  Port=4
  Bus Creator : BusCreator  Inputs=4
  Bus Creator1 : BusCreator  Inputs=3
  Bus Creator2 : BusCreator  Inputs=3
  Bus Selector1 : BusSelector  OutputSignals=Range,Speed,Gain
  Constant : Constant  Value=77.0
  Constant1 : Constant  Value=1.0
  Constant11 : Constant  Value=0.0
  Constant12 : Constant  Value=0.0
  Constant2 : Constant  Value=0.52
  Constant3 : Constant  Value=13.0
  Constant4 : Constant  Value=13.0
  Constant5 : Constant  Value=0.3
  Constant6 : Constant  Value=0.0
  DARTS Eth : dsmpblib/Data Inport  Priority=10000
      settings: SourceProductName=dSPACE Model Interface Package for Simulink (MIPS)
  Demux : Demux  Outputs=3
  Demux1 : Demux  Outputs=3
  Ground : Ground
  Mux1 : Mux  Inputs=3
  Mux2 : Mux  Inputs=3
  Setup Status [DARTS Control (1)] : dsmpblib/Data Inport  Priority=10000
      settings: SourceProductName=dSPACE Model Interface Package for Simulink (MIPS)
  Setup [DARTS Control (1)] : dsmpblib/Data Outport  Priority=-10000
      settings: SourceProductName=dSPACE Model Interface Package for Simulink (MIPS)
  Status [DARTS Control (1)] : dsmpblib/Data Inport  Priority=10000
      settings: SourceProductName=dSPACE Model Interface Package for Simulink (MIPS)
  Targets Status [DARTS Control (1)] : dsmpblib/Data Inport  Priority=10000
      settings: SourceProductName=dSPACE Model Interface Package for Simulink (MIPS)
  Targets [DARTS Control (1)] : dsmpblib/Data Outport  Priority=-10000
      settings: SourceProductName=dSPACE Model Interface Package for Simulink (MIPS)
  Terminator{1..17} (17 alike) : Terminator
  Trigger [DARTS Control (1)] : dsmpblib/Data Outport  Priority=-10000
      settings: SourceProductName=dSPACE Model Interface Package for Simulink (MIPS)
  tag scope: dartsInput=global, dartsResponse=global
  wires:
  Setup Status [DARTS Control (1)]/9 -> Terminator10/1
  Ground/1 -> Trigger [DARTS Control (1)]/3, Trigger [DARTS Control (1)]/2, Trigger [DARTS Control (1)]/1
  Setup Status [DARTS Control (1)]/2 -> Terminator3/1
  Setup Status [DARTS Control (1)]/8 -> Terminator9/1
  Setup Status [DARTS Control (1)]/3 -> Terminator4/1
  Status [DARTS Control (1)]/1 -> Terminator11/1
  Setup Status [DARTS Control (1)]/6 -> Terminator7/1
  Setup Status [DARTS Control (1)]/5 -> Terminator6/1
  Setup Status [DARTS Control (1)]/7 -> Terminator8/1
  Setup Status [DARTS Control (1)]/4 -> Terminator5/1
  Status [DARTS Control (1)]/7 -> Terminator16/1
  Setup Status [DARTS Control (1)]/1 -> Terminator2/1
  Demux1/3 -> Bus Creator2/3  "OutGain"
  Status [DARTS Control (1)]/4 -> Terminator17/1
  Status [DARTS Control (1)]/5 -> Terminator14/1
  Bus Selector1/3 -> Mux2/3  "<Gain>"
  Status [DARTS Control (1)]/6 -> Terminator15/1
  Status [DARTS Control (1)]/2 -> Terminator12/1
  Constant11/1 -> Setup [DARTS Control (1)]/6
  Status [DARTS Control (1)]/3 -> Terminator13/1
  Mux2/1 -> Demux1/1
  Demux1/2 -> Bus Creator2/2  "OutSpeed"
  Demux1/1 -> Bus Creator2/1  "OutRange"
  Bus Selector1/2 -> Mux2/2  "<Speed>"
  Constant12/1 -> Setup [DARTS Control (1)]/2
  Constant/1 -> Setup [DARTS Control (1)]/1
  Bus Creator2/1 -> [dartsResponse]
  Constant4/1 -> Setup [DARTS Control (1)]/9
  Constant1/1 -> Setup [DARTS Control (1)]/5
  Constant6/1 -> Setup [DARTS Control (1)]/3
  Bus Selector1/1 -> Mux2/1  "<Range>"
  Constant2/1 -> Setup [DARTS Control (1)]/4
  DARTS Eth/1 -> Terminator1/1
  Constant3/1 -> Setup [DARTS Control (1)]/8
  Targets Status [DARTS Control (1)]/1 -> Bus Selector1/1
  Constant5/1 -> Setup [DARTS Control (1)]/7
  Demux/1 -> Bus Creator1/1  "InRange"
  Mux1/1 -> Demux/1
  Demux/3 -> Bus Creator1/3  "InGain"
  Bus Creator/1 -> Targets [DARTS Control (1)]/1
  Demux/2 -> Bus Creator1/2  "InSpeed"
  Bus Creator1/1 -> [dartsInput]
  Enable/1 -> Bus Creator/1  "Enable"
  Range/1 -> Mux1/1, Bus Creator/2  "Range"
  Speed/1 -> Mux1/2, Bus Creator/3  "Speed"
  Gain/1 -> Mux1/3, Bus Creator/4  "Gain"
